simulink model "half_adder"  (R2015a)
settings: Solver=ode23t  StartTime=0.0  StopTime=10  RelTol=1e-3
libraries: fl_lib x115, nesl_utility x109, elec_lib x10
(part 2 of 2)

== system half_adder/AND/DCM2/DCM/Memristor3 ==
  Current Sensor : fl_lib/Electrical/Electrical Sensors/Current Sensor
  Fcn : Fcn  Expr=1-(u-1)^(2*10)
  Fcn1 : Fcn  Expr=16e3-u*(15.9e3)
  Gain : Gain  Gain=1e4
  Integrator : Integrator  InitialCondition=rand()
  PS-Simulink Converter : nesl_utility/PS-Simulink Converter  PhysicalDomain=network_engine_domain  SubClassName=ps_output  LeftPortType=input  RightPortType=output  PseudoPeriodic=off  Frequencies=[]  Unit=1  AffineConversion=off
  Product : Product
  Simulink-PS Converter : nesl_utility/Simulink-PS Converter  PhysicalDomain=network_engine_domain  SubClassName=ps_input  LeftPortType=input  RightPortType=output  PseudoPeriodic=off  Frequencies=[]  NoiseDistribution=none  NoiseParameters=[]  Unit=1  AffineConversion=off  InputFiltering=off  SimscapeFilterOrder=1  InputFilterTimeConstant=0.001  UdotUserProvided=1
  Variable Resistor : fl_lib/Electrical/Electrical Elements/Variable Resistor  Rmin=100 Ohm  i_specify=off  i_priority=High  i=0 A  v_specify=off  v_priority=High  v=0 V
  In : PMIOPort  Port=1  Side=Left
  Out : PMIOPort  Port=2  Side=Right
  wires:
  Gain/1 -> Integrator/1
  Product/1 -> Gain/1
  Integrator/1 -> Fcn1/1, Fcn/1
  Fcn/1 -> Product/2
  Fcn1/1 -> Simulink-PS Converter/1
  PS-Simulink Converter/1 -> Product/1
  connections:
  Current Sensor/RConn1 -- PS-Simulink Converter/LConn1
  Current Sensor/RConn2 -- Out/RConn1
  Variable Resistor/LConn2 -- In/RConn1
  Simulink-PS Converter/RConn1 -- Variable Resistor/LConn1
  Variable Resistor/RConn1 -- Current Sensor/LConn1

== system half_adder/XOR/DCM/DCM/Memristor ==
  Current Sensor : fl_lib/Electrical/Electrical Sensors/Current Sensor
  Fcn : Fcn  Expr=1-(u-1)^(2*10)
  Fcn1 : Fcn  Expr=16e3-u*(15.9e3)
  Gain : Gain  Gain=1e4
  Integrator : Integrator  InitialCondition=rand()
  PS-Simulink Converter : nesl_utility/PS-Simulink Converter  PhysicalDomain=network_engine_domain  SubClassName=ps_output  LeftPortType=input  RightPortType=output  PseudoPeriodic=off  Frequencies=[]  Unit=1  AffineConversion=off
  Product : Product
  Scope : Scope
  Simulink-PS Converter : nesl_utility/Simulink-PS Converter  PhysicalDomain=network_engine_domain  SubClassName=ps_input  LeftPortType=input  RightPortType=output  PseudoPeriodic=off  Frequencies=[]  NoiseDistribution=none  NoiseParameters=[]  Unit=1  AffineConversion=off  InputFiltering=off  SimscapeFilterOrder=1  InputFilterTimeConstant=0.001  UdotUserProvided=1
  Variable Resistor : fl_lib/Electrical/Electrical Elements/Variable Resistor  Rmin=100 Ohm  i_specify=off  i_priority=High  i=0 A  v_specify=off  v_priority=High  v=0 V
  In : PMIOPort  Port=1  Side=Left
  Out : PMIOPort  Port=2  Side=Right
  wires:
  Gain/1 -> Integrator/1
  Product/1 -> Gain/1
  Integrator/1 -> Scope/1, Fcn1/1, Fcn/1
  Fcn/1 -> Product/2
  Fcn1/1 -> Simulink-PS Converter/1
  PS-Simulink Converter/1 -> Product/1
  connections:
  Current Sensor/RConn1 -- PS-Simulink Converter/LConn1
  Simulink-PS Converter/RConn1 -- Variable Resistor/LConn1
  Current Sensor/RConn2 -- Out/RConn1
  Variable Resistor/RConn1 -- Current Sensor/LConn1
  Variable Resistor/LConn2 -- In/RConn1

== system half_adder/XOR/DCM/DCM/Memristor1 ==
  Current Sensor : fl_lib/Electrical/Electrical Sensors/Current Sensor
  Fcn : Fcn  Expr=1-(u-1)^(2*10)
  Fcn1 : Fcn  Expr=16e3-u*(15.9e3)
  Gain : Gain  Gain=1e4
  Integrator : Integrator  InitialCondition=rand()
  PS-Simulink Converter : nesl_utility/PS-Simulink Converter  PhysicalDomain=network_engine_domain  SubClassName=ps_output  LeftPortType=input  RightPortType=output  PseudoPeriodic=off  Frequencies=[]  Unit=1  AffineConversion=off
  Product : Product
  Simulink-PS Converter : nesl_utility/Simulink-PS Converter  PhysicalDomain=network_engine_domain  SubClassName=ps_input  LeftPortType=input  RightPortType=output  PseudoPeriodic=off  Frequencies=[]  NoiseDistribution=none  NoiseParameters=[]  Unit=1  AffineConversion=off  InputFiltering=off  SimscapeFilterOrder=1  InputFilterTimeConstant=0.001  UdotUserProvided=1
  Variable Resistor : fl_lib/Electrical/Electrical Elements/Variable Resistor  Rmin=100 Ohm  i_specify=off  i_priority=High  i=0 A  v_specify=off  v_priority=High  v=0 V
  In : PMIOPort  Port=1  Side=Left
  Out : PMIOPort  Port=2  Side=Right
  wires:
  Gain/1 -> Integrator/1
  Product/1 -> Gain/1
  Integrator/1 -> Fcn1/1, Fcn/1
  Fcn/1 -> Product/2
  Fcn1/1 -> Simulink-PS Converter/1
  PS-Simulink Converter/1 -> Product/1
  connections:
  Variable Resistor/LConn2 -- In/RConn1
  Current Sensor/RConn1 -- PS-Simulink Converter/LConn1
  Current Sensor/RConn2 -- Out/RConn1
  Simulink-PS Converter/RConn1 -- Variable Resistor/LConn1
  Variable Resistor/RConn1 -- Current Sensor/LConn1

== system half_adder/XOR/DCM/DCM/Memristor2 ==
  Current Sensor : fl_lib/Electrical/Electrical Sensors/Current Sensor
  Fcn : Fcn  Expr=1-(u-1)^(2*10)
  Fcn1 : Fcn  Expr=16e3-u*(15.9e3)
  Gain : Gain  Gain=1e4
  Integrator : Integrator  InitialCondition=rand()
  PS-Simulink Converter : nesl_utility/PS-Simulink Converter  PhysicalDomain=network_engine_domain  SubClassName=ps_output  LeftPortType=input  RightPortType=output  PseudoPeriodic=off  Frequencies=[]  Unit=1  AffineConversion=off
  Product : Product
  Simulink-PS Converter : nesl_utility/Simulink-PS Converter  PhysicalDomain=network_engine_domain  SubClassName=ps_input  LeftPortType=input  RightPortType=output  PseudoPeriodic=off  Frequencies=[]  NoiseDistribution=none  NoiseParameters=[]  Unit=1  AffineConversion=off  InputFiltering=off  SimscapeFilterOrder=1  InputFilterTimeConstant=0.001  UdotUserProvided=1
  Variable Resistor : fl_lib/Electrical/Electrical Elements/Variable Resistor  Rmin=100 Ohm  i_specify=off  i_priority=High  i=0 A  v_specify=off  v_priority=High  v=0 V
  In : PMIOPort  Port=1  Side=Left
  Out : PMIOPort  Port=2  Side=Right
  wires:
  Gain/1 -> Integrator/1
  Product/1 -> Gain/1
  Integrator/1 -> Fcn1/1, Fcn/1
  Fcn/1 -> Product/2
  Fcn1/1 -> Simulink-PS Converter/1
  PS-Simulink Converter/1 -> Product/1
  connections:
  Variable Resistor/LConn2 -- In/RConn1
  Current Sensor/RConn1 -- PS-Simulink Converter/LConn1
  Current Sensor/RConn2 -- Out/RConn1
  Variable Resistor/RConn1 -- Current Sensor/LConn1
  Simulink-PS Converter/RConn1 -- Variable Resistor/LConn1

== system half_adder/XOR/DCM/DCM/Memristor3 ==
  Current Sensor : fl_lib/Electrical/Electrical Sensors/Current Sensor
  Fcn : Fcn  Expr=1-(u-1)^(2*10)
  Fcn1 : Fcn  Expr=16e3-u*(15.9e3)
  Gain : Gain  Gain=1e4
  Integrator : Integrator  InitialCondition=rand()
  PS-Simulink Converter : nesl_utility/PS-Simulink Converter  PhysicalDomain=network_engine_domain  SubClassName=ps_output  LeftPortType=input  RightPortType=output  PseudoPeriodic=off  Frequencies=[]  Unit=1  AffineConversion=off
  Product : Product
  Simulink-PS Converter : nesl_utility/Simulink-PS Converter  PhysicalDomain=network_engine_domain  SubClassName=ps_input  LeftPortType=input  RightPortType=output  PseudoPeriodic=off  Frequencies=[]  NoiseDistribution=none  NoiseParameters=[]  Unit=1  AffineConversion=off  InputFiltering=off  SimscapeFilterOrder=1  InputFilterTimeConstant=0.001  UdotUserProvided=1
  Variable Resistor : fl_lib/Electrical/Electrical Elements/Variable Resistor  Rmin=100 Ohm  i_specify=off  i_priority=High  i=0 A  v_specify=off  v_priority=High  v=0 V
  In : PMIOPort  Port=1  Side=Left
  Out : PMIOPort  Port=2  Side=Right
  wires:
  Gain/1 -> Integrator/1
  Product/1 -> Gain/1
  Integrator/1 -> Fcn1/1, Fcn/1
  Fcn/1 -> Product/2
  Fcn1/1 -> Simulink-PS Converter/1
  PS-Simulink Converter/1 -> Product/1
  connections:
  Current Sensor/RConn1 -- PS-Simulink Converter/LConn1
  Current Sensor/RConn2 -- Out/RConn1
  Variable Resistor/LConn2 -- In/RConn1
  Simulink-PS Converter/RConn1 -- Variable Resistor/LConn1
  Variable Resistor/RConn1 -- Current Sensor/LConn1

== system half_adder/XOR/DCM1/DCM/Memristor ==
  Current Sensor : fl_lib/Electrical/Electrical Sensors/Current Sensor
  Fcn : Fcn  Expr=1-(u-1)^(2*10)
  Fcn1 : Fcn  Expr=16e3-u*(15.9e3)
  Gain : Gain  Gain=1e4
  Integrator : Integrator  InitialCondition=rand()
  PS-Simulink Converter : nesl_utility/PS-Simulink Converter  PhysicalDomain=network_engine_domain  SubClassName=ps_output  LeftPortType=input  RightPortType=output  PseudoPeriodic=off  Frequencies=[]  Unit=1  AffineConversion=off
  Product : Product
  Scope : Scope
  Simulink-PS Converter : nesl_utility/Simulink-PS Converter  PhysicalDomain=network_engine_domain  SubClassName=ps_input  LeftPortType=input  RightPortType=output  PseudoPeriodic=off  Frequencies=[]  NoiseDistribution=none  NoiseParameters=[]  Unit=1  AffineConversion=off  InputFiltering=off  SimscapeFilterOrder=1  InputFilterTimeConstant=0.001  UdotUserProvided=1
  Variable Resistor : fl_lib/Electrical/Electrical Elements/Variable Resistor  Rmin=100 Ohm  i_specify=off  i_priority=High  i=0 A  v_specify=off  v_priority=High  v=0 V
  In : PMIOPort  Port=1  Side=Left
  Out : PMIOPort  Port=2  Side=Right
  wires:
  Gain/1 -> Integrator/1
  Product/1 -> Gain/1
  Integrator/1 -> Scope/1, Fcn1/1, Fcn/1
  Fcn/1 -> Product/2
  Fcn1/1 -> Simulink-PS Converter/1
  PS-Simulink Converter/1 -> Product/1
  connections:
  Current Sensor/RConn1 -- PS-Simulink Converter/LConn1
  Simulink-PS Converter/RConn1 -- Variable Resistor/LConn1
  Current Sensor/RConn2 -- Out/RConn1
  Variable Resistor/RConn1 -- Current Sensor/LConn1
  Variable Resistor/LConn2 -- In/RConn1

== system half_adder/XOR/DCM1/DCM/Memristor1 ==
  Current Sensor : fl_lib/Electrical/Electrical Sensors/Current Sensor
  Fcn : Fcn  Expr=1-(u-1)^(2*10)
  Fcn1 : Fcn  Expr=16e3-u*(15.9e3)
  Gain : Gain  Gain=1e4
  Integrator : Integrator  InitialCondition=rand()
  PS-Simulink Converter : nesl_utility/PS-Simulink Converter  PhysicalDomain=network_engine_domain  SubClassName=ps_output  LeftPortType=input  RightPortType=output  PseudoPeriodic=off  Frequencies=[]  Unit=1  AffineConversion=off
  Product : Product
  Simulink-PS Converter : nesl_utility/Simulink-PS Converter  PhysicalDomain=network_engine_domain  SubClassName=ps_input  LeftPortType=input  RightPortType=output  PseudoPeriodic=off  Frequencies=[]  NoiseDistribution=none  NoiseParameters=[]  Unit=1  AffineConversion=off  InputFiltering=off  SimscapeFilterOrder=1  InputFilterTimeConstant=0.001  UdotUserProvided=1
  Variable Resistor : fl_lib/Electrical/Electrical Elements/Variable Resistor  Rmin=100 Ohm  i_specify=off  i_priority=High  i=0 A  v_specify=off  v_priority=High  v=0 V
  In : PMIOPort  Port=1  Side=Left
  Out : PMIOPort  Port=2  Side=Right
  wires:
  Gain/1 -> Integrator/1
  Product/1 -> Gain/1
  Integrator/1 -> Fcn1/1, Fcn/1
  Fcn/1 -> Product/2
  Fcn1/1 -> Simulink-PS Converter/1
  PS-Simulink Converter/1 -> Product/1
  connections:
  Variable Resistor/LConn2 -- In/RConn1
  Current Sensor/RConn1 -- PS-Simulink Converter/LConn1
  Current Sensor/RConn2 -- Out/RConn1
  Simulink-PS Converter/RConn1 -- Variable Resistor/LConn1
  Variable Resistor/RConn1 -- Current Sensor/LConn1

== system half_adder/XOR/DCM1/DCM/Memristor2 ==
  Current Sensor : fl_lib/Electrical/Electrical Sensors/Current Sensor
  Fcn : Fcn  Expr=1-(u-1)^(2*10)
  Fcn1 : Fcn  Expr=16e3-u*(15.9e3)
  Gain : Gain  Gain=1e4
  Integrator : Integrator  InitialCondition=rand()
  PS-Simulink Converter : nesl_utility/PS-Simulink Converter  PhysicalDomain=network_engine_domain  SubClassName=ps_output  LeftPortType=input  RightPortType=output  PseudoPeriodic=off  Frequencies=[]  Unit=1  AffineConversion=off
  Product : Product
  Simulink-PS Converter : nesl_utility/Simulink-PS Converter  PhysicalDomain=network_engine_domain  SubClassName=ps_input  LeftPortType=input  RightPortType=output  PseudoPeriodic=off  Frequencies=[]  NoiseDistribution=none  NoiseParameters=[]  Unit=1  AffineConversion=off  InputFiltering=off  SimscapeFilterOrder=1  InputFilterTimeConstant=0.001  UdotUserProvided=1
  Variable Resistor : fl_lib/Electrical/Electrical Elements/Variable Resistor  Rmin=100 Ohm  i_specify=off  i_priority=High  i=0 A  v_specify=off  v_priority=High  v=0 V
  In : PMIOPort  Port=1  Side=Left
  Out : PMIOPort  Port=2  Side=Right
  wires:
  Gain/1 -> Integrator/1
  Product/1 -> Gain/1
  Integrator/1 -> Fcn1/1, Fcn/1
  Fcn/1 -> Product/2
  Fcn1/1 -> Simulink-PS Converter/1
  PS-Simulink Converter/1 -> Product/1
  connections:
  Variable Resistor/LConn2 -- In/RConn1
  Current Sensor/RConn1 -- PS-Simulink Converter/LConn1
  Current Sensor/RConn2 -- Out/RConn1
  Variable Resistor/RConn1 -- Current Sensor/LConn1
  Simulink-PS Converter/RConn1 -- Variable Resistor/LConn1

== system half_adder/XOR/DCM1/DCM/Memristor3 ==
  Current Sensor : fl_lib/Electrical/Electrical Sensors/Current Sensor
  Fcn : Fcn  Expr=1-(u-1)^(2*10)
  Fcn1 : Fcn  Expr=16e3-u*(15.9e3)
  Gain : Gain  Gain=1e4
  Integrator : Integrator  InitialCondition=rand()
  PS-Simulink Converter : nesl_utility/PS-Simulink Converter  PhysicalDomain=network_engine_domain  SubClassName=ps_output  LeftPortType=input  RightPortType=output  PseudoPeriodic=off  Frequencies=[]  Unit=1  AffineConversion=off
  Product : Product
  Simulink-PS Converter : nesl_utility/Simulink-PS Converter  PhysicalDomain=network_engine_domain  SubClassName=ps_input  LeftPortType=input  RightPortType=output  PseudoPeriodic=off  Frequencies=[]  NoiseDistribution=none  NoiseParameters=[]  Unit=1  AffineConversion=off  InputFiltering=off  SimscapeFilterOrder=1  InputFilterTimeConstant=0.001  UdotUserProvided=1
  Variable Resistor : fl_lib/Electrical/Electrical Elements/Variable Resistor  Rmin=100 Ohm  i_specify=off  i_priority=High  i=0 A  v_specify=off  v_priority=High  v=0 V
  In : PMIOPort  Port=1  Side=Left
  Out : PMIOPort  Port=2  Side=Right
  wires:
  Gain/1 -> Integrator/1
  Product/1 -> Gain/1
  Integrator/1 -> Fcn1/1, Fcn/1
  Fcn/1 -> Product/2
  Fcn1/1 -> Simulink-PS Converter/1
  PS-Simulink Converter/1 -> Product/1
  connections:
  Current Sensor/RConn1 -- PS-Simulink Converter/LConn1
  Current Sensor/RConn2 -- Out/RConn1
  Variable Resistor/LConn2 -- In/RConn1
  Simulink-PS Converter/RConn1 -- Variable Resistor/LConn1
  Variable Resistor/RConn1 -- Current Sensor/LConn1

== system half_adder/XOR/DCM2/DCM/Memristor ==
  Current Sensor : fl_lib/Electrical/Electrical Sensors/Current Sensor
  Fcn : Fcn  Expr=1-(u-1)^(2*10)
  Fcn1 : Fcn  Expr=16e3-u*(15.9e3)
  Gain : Gain  Gain=1e4
  Integrator : Integrator  InitialCondition=rand()
  PS-Simulink Converter : nesl_utility/PS-Simulink Converter  PhysicalDomain=network_engine_domain  SubClassName=ps_output  LeftPortType=input  RightPortType=output  PseudoPeriodic=off  Frequencies=[]  Unit=1  AffineConversion=off
  Product : Product
  Scope : Scope
  Simulink-PS Converter : nesl_utility/Simulink-PS Converter  PhysicalDomain=network_engine_domain  SubClassName=ps_input  LeftPortType=input  RightPortType=output  PseudoPeriodic=off  Frequencies=[]  NoiseDistribution=none  NoiseParameters=[]  Unit=1  AffineConversion=off  InputFiltering=off  SimscapeFilterOrder=1  InputFilterTimeConstant=0.001  UdotUserProvided=1
  Variable Resistor : fl_lib/Electrical/Electrical Elements/Variable Resistor  Rmin=100 Ohm  i_specify=off  i_priority=High  i=0 A  v_specify=off  v_priority=High  v=0 V
  In : PMIOPort  Port=1  Side=Left
  Out : PMIOPort  Port=2  Side=Right
  wires:
  Gain/1 -> Integrator/1
  Product/1 -> Gain/1
  Integrator/1 -> Scope/1, Fcn1/1, Fcn/1
  Fcn/1 -> Product/2
  Fcn1/1 -> Simulink-PS Converter/1
  PS-Simulink Converter/1 -> Product/1
  connections:
  Current Sensor/RConn1 -- PS-Simulink Converter/LConn1
  Simulink-PS Converter/RConn1 -- Variable Resistor/LConn1
  Current Sensor/RConn2 -- Out/RConn1
  Variable Resistor/RConn1 -- Current Sensor/LConn1
  Variable Resistor/LConn2 -- In/RConn1

== system half_adder/XOR/DCM2/DCM/Memristor1 ==
  Current Sensor : fl_lib/Electrical/Electrical Sensors/Current Sensor
  Fcn : Fcn  Expr=1-(u-1)^(2*10)
  Fcn1 : Fcn  Expr=16e3-u*(15.9e3)
  Gain : Gain  Gain=1e4
  Integrator : Integrator  InitialCondition=rand()
  PS-Simulink Converter : nesl_utility/PS-Simulink Converter  PhysicalDomain=network_engine_domain  SubClassName=ps_output  LeftPortType=input  RightPortType=output  PseudoPeriodic=off  Frequencies=[]  Unit=1  AffineConversion=off
  Product : Product
  Simulink-PS Converter : nesl_utility/Simulink-PS Converter  PhysicalDomain=network_engine_domain  SubClassName=ps_input  LeftPortType=input  RightPortType=output  PseudoPeriodic=off  Frequencies=[]  NoiseDistribution=none  NoiseParameters=[]  Unit=1  AffineConversion=off  InputFiltering=off  SimscapeFilterOrder=1  InputFilterTimeConstant=0.001  UdotUserProvided=1
  Variable Resistor : fl_lib/Electrical/Electrical Elements/Variable Resistor  Rmin=100 Ohm  i_specify=off  i_priority=High  i=0 A  v_specify=off  v_priority=High  v=0 V
  In : PMIOPort  Port=1  Side=Left
  Out : PMIOPort  Port=2  Side=Right
  wires:
  Gain/1 -> Integrator/1
  Product/1 -> Gain/1
  Integrator/1 -> Fcn1/1, Fcn/1
  Fcn/1 -> Product/2
  Fcn1/1 -> Simulink-PS Converter/1
  PS-Simulink Converter/1 -> Product/1
  connections:
  Variable Resistor/LConn2 -- In/RConn1
  Current Sensor/RConn1 -- PS-Simulink Converter/LConn1
  Current Sensor/RConn2 -- Out/RConn1
  Simulink-PS Converter/RConn1 -- Variable Resistor/LConn1
  Variable Resistor/RConn1 -- Current Sensor/LConn1

== system half_adder/XOR/DCM2/DCM/Memristor2 ==
  Current Sensor : fl_lib/Electrical/Electrical Sensors/Current Sensor
  Fcn : Fcn  Expr=1-(u-1)^(2*10)
  Fcn1 : Fcn  Expr=16e3-u*(15.9e3)
  Gain : Gain  Gain=1e4
  Integrator : Integrator  InitialCondition=rand()
  PS-Simulink Converter : nesl_utility/PS-Simulink Converter  PhysicalDomain=network_engine_domain  SubClassName=ps_output  LeftPortType=input  RightPortType=output  PseudoPeriodic=off  Frequencies=[]  Unit=1  AffineConversion=off
  Product : Product
  Simulink-PS Converter : nesl_utility/Simulink-PS Converter  PhysicalDomain=network_engine_domain  SubClassName=ps_input  LeftPortType=input  RightPortType=output  PseudoPeriodic=off  Frequencies=[]  NoiseDistribution=none  NoiseParameters=[]  Unit=1  AffineConversion=off  InputFiltering=off  SimscapeFilterOrder=1  InputFilterTimeConstant=0.001  UdotUserProvided=1
  Variable Resistor : fl_lib/Electrical/Electrical Elements/Variable Resistor  Rmin=100 Ohm  i_specify=off  i_priority=High  i=0 A  v_specify=off  v_priority=High  v=0 V
  In : PMIOPort  Port=1  Side=Left
  Out : PMIOPort  Port=2  Side=Right
  wires:
  Gain/1 -> Integrator/1
  Product/1 -> Gain/1
  Integrator/1 -> Fcn1/1, Fcn/1
  Fcn/1 -> Product/2
  Fcn1/1 -> Simulink-PS Converter/1
  PS-Simulink Converter/1 -> Product/1
  connections:
  Variable Resistor/LConn2 -- In/RConn1
  Current Sensor/RConn1 -- PS-Simulink Converter/LConn1
  Current Sensor/RConn2 -- Out/RConn1
  Variable Resistor/RConn1 -- Current Sensor/LConn1
  Simulink-PS Converter/RConn1 -- Variable Resistor/LConn1

== system half_adder/XOR/DCM2/DCM/Memristor3 ==
  Current Sensor : fl_lib/Electrical/Electrical Sensors/Current Sensor
  Fcn : Fcn  Expr=1-(u-1)^(2*10)
  Fcn1 : Fcn  Expr=16e3-u*(15.9e3)
  Gain : Gain  Gain=1e4
  Integrator : Integrator  InitialCondition=rand()
  PS-Simulink Converter : nesl_utility/PS-Simulink Converter  PhysicalDomain=network_engine_domain  SubClassName=ps_output  LeftPortType=input  RightPortType=output  PseudoPeriodic=off  Frequencies=[]  Unit=1  AffineConversion=off
  Product : Product
  Simulink-PS Converter : nesl_utility/Simulink-PS Converter  PhysicalDomain=network_engine_domain  SubClassName=ps_input  LeftPortType=input  RightPortType=output  PseudoPeriodic=off  Frequencies=[]  NoiseDistribution=none  NoiseParameters=[]  Unit=1  AffineConversion=off  InputFiltering=off  SimscapeFilterOrder=1  InputFilterTimeConstant=0.001  UdotUserProvided=1
  Variable Resistor : fl_lib/Electrical/Electrical Elements/Variable Resistor  Rmin=100 Ohm  i_specify=off  i_priority=High  i=0 A  v_specify=off  v_priority=High  v=0 V
  In : PMIOPort  Port=1  Side=Left
  Out : PMIOPort  Port=2  Side=Right
  wires:
  Gain/1 -> Integrator/1
  Product/1 -> Gain/1
  Integrator/1 -> Fcn1/1, Fcn/1
  Fcn/1 -> Product/2
  Fcn1/1 -> Simulink-PS Converter/1
  PS-Simulink Converter/1 -> Product/1
  connections:
  Current Sensor/RConn1 -- PS-Simulink Converter/LConn1
  Current Sensor/RConn2 -- Out/RConn1
  Variable Resistor/LConn2 -- In/RConn1
  Simulink-PS Converter/RConn1 -- Variable Resistor/LConn1
  Variable Resistor/RConn1 -- Current Sensor/LConn1
